simulink model "finc_call1"  (Simulink 4.00)
settings: Solver=ode45  StartTime=0.0  StopTime=30.0  RelTol=1e-3
settings Model: LastModifiedBy=Administrator  BlockReductionOpt=off

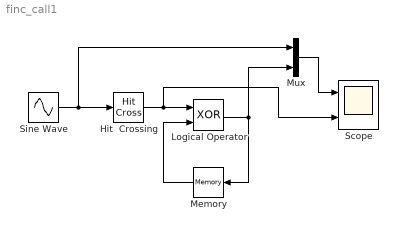
== system finc_call1 ==
  Hit  Crossing : HitCross  HitCrossingOffset=0  HitCrossingDirection=rising  ShowOutputPort=on
  Logical Operator : Logic  Operator=XOR  Inputs=2
  Memory : Memory  Orientation=left  X0=0  InheritSampleTime=off
  Mux : Mux  Inputs=2
  Scope : Scope  NumInputPorts=2
      settings: TimeRange=auto  YMin=-5~-5  YMax=5~5  SaveToWorkspace=off  SaveName=ScopeData  LimitDataPoints=on  MaxDataPoints=5000
  Sine Wave : Sin  Amplitude=1  Frequency=1  Phase=0  SampleTime=0
  wires:
  Sine Wave/1 -> Hit  Crossing/1, Mux/1
  Hit  Crossing/1 -> Logical Operator/1, Scope/2
  Memory/1 -> Logical Operator/2
  Logical Operator/1 -> Memory/1, Mux/2
  Mux/1 -> Scope/1
